simulink model "vehicle_model_cfeng"  (R2024b)
settings: Solver=FixedStepAuto  StartTime=0.0  StopTime=500.0  FixedStep=ts  RelTol=1e-3
InitFcn:
  | vehicle_parameter_Mercedes_A180
values from neighbouring files (symbols this model uses):
  acc_motor = [0, 0.13, 6.25, 12.5, 18.75, 25, 31.25, 37.5, 43.75, 50, 56.25, 62.5, 68.75, 75, 81.25, 90.63, 100]    [vehicle_parameter_Mercedes_A180.m]
  c_whl = 2 * pi * r_whl    (= 2.0106192983)    [vehicle_parameter_Mercedes_A180.m]
  eng_trq = [0, 25, 50, 75, 100, 125, 150, 175, 200, 225, 250, 275, 300]    [vehicle_parameter_Mercedes_A180.m]
  g = 9.81    [vehicle_parameter_Mercedes_A180.m]
  gear_ratios_to_neutral = [1, 1.0526, 1.1368, 1.2421, 1.3263, 1.4737, 1.6421, 1.1895]    [vehicle_parameter_Mercedes_A180.m]
  i_brems = 12    [vehicle_parameter_Mercedes_A180.m]
  m_tot = m_veh + m_pay    (= 1445)    [vehicle_parameter_Mercedes_A180.m]
  mu_brems = 0.8    [vehicle_parameter_Mercedes_A180.m]
  n_brems = 2    [vehicle_parameter_Mercedes_A180.m]
  r_air = cw_drag * A_face    (= 0.594)    [vehicle_parameter_Mercedes_A180.m]
  r_axle = 3.35    [vehicle_parameter_Mercedes_A180.m]
  r_brems = 0.1    [vehicle_parameter_Mercedes_A180.m]
  r_gear = [0.00, 4.31, 2.44, 1.35, 0.94, 0.82, 0.70, 3.38]    [vehicle_parameter_Mercedes_A180.m]
  r_roll = 0.0125    [vehicle_parameter_Mercedes_A180.m]
  r_whl = 0.32    [vehicle_parameter_Mercedes_A180.m]
  roh_air = 1.204    [vehicle_parameter_Mercedes_A180.m]
  rpm_drag = [0, 1, 500, 1000, 1500, 2000, 2500, 3000, 3500, 4000, 4500, 5000, 5500]    [vehicle_parameter_Mercedes_A180.m]
  rpm_loss = [0, 500, 1000, 1500, 2000, 2500, 3000, 3500, 4000, 4500, 5000, 5500]    [vehicle_parameter_Mercedes_A180.m]
  rpm_motor = [0, 608, 640, 736, 800, 992, 1248, 1504, 1760, 2016, 2240, 2496, 2752, 3008, 3264, 3488, 3744, 4000, 4512, 4992, 5248, 5500]    [vehicle_parameter_Mercedes_A180.m]
  torque_drag = [0, 10.27, 10.53, 10.93, 11.46, 12.12, 12.91, 13.84, 14.90, 16.09, 17.41, 18.86, 20.45]    [vehicle_parameter_Mercedes_A180.m]
  torque_loss = [ ... (first row only)    [vehicle_parameter_Mercedes_A180.m]
  torque_motor = [ ... (first row only)    [vehicle_parameter_Mercedes_A180.m]
undefined symbols (not defined in the file or in its folder): magnitude
libraries: simulink x4, slpidlib x1
settings Model: Creator=ASUS  LastModifiedBy=ASUS
settings RTWCC: GPUComputeCapability=3.5

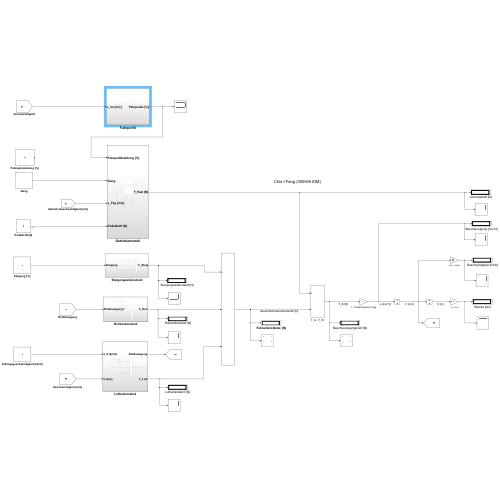
[thumbnail: Simulink's stored preview of the top-level diagram]
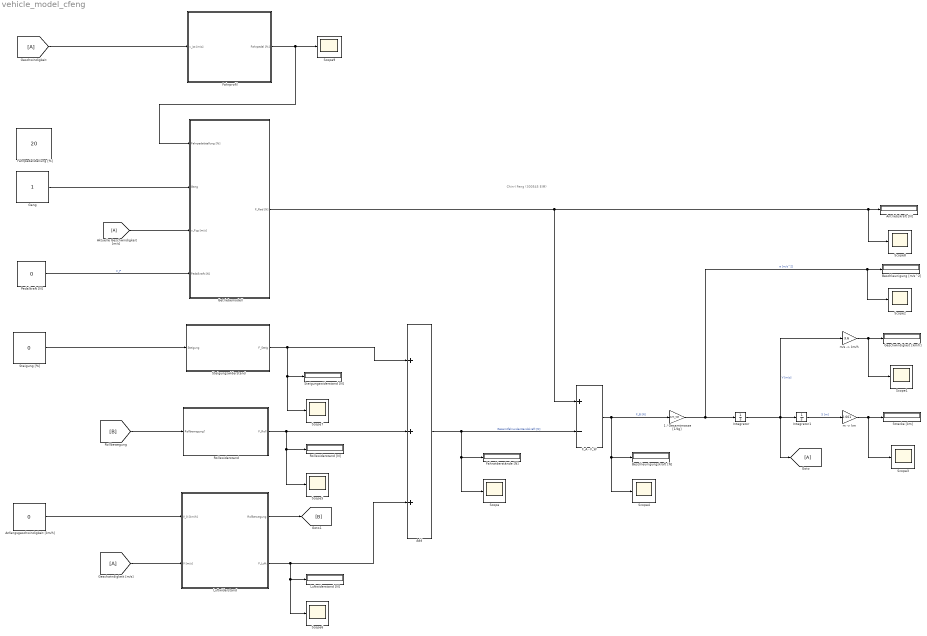
== system vehicle_model_cfeng ==
  note: Chin-I Feng (300545 EIM)
  1 / Gesamtmasse [1/kg] : Gain  Gain=1/m_tot
  Add : Sum  Inputs=+++
  Aktuelle Geschwindigkeit [m/s] : From
  Anfangsgeschwindigkeit [km/h] : Constant  Value=0  SampleTime=1
  Antriebskraft [N] : Display
  Beschleunigung [m/s^2] : Display
  Beschleunigungskraft [N] : Display
  F_A - F_W : Sum  Inputs=+-
  Fahrpedalstellung [%] : Constant  Value=20  SampleTime=1
  Fahrprofil : Subsystem
  Fahrwiderstände [N] : Display
  Gang : Constant  SampleTime=1
  Geschwindigkeit : From
  Geschwindigkeit [km/h] : Display
  Geschwindigkeit [m/s] : From
  Getriebemodell : Subsystem
  Goto : Goto
  Integrator : Integrator
  Integrator1 : Integrator
  Luftwiderstand : Subsystem
  "Luftwiderstand [N] " : Display
  Pedalkraft [N] : Constant  Value=0  SampleTime=1
  Rollswiderstand : Subsystem
  Rollswiderstand [N] : Display
  Scope{,1..9} (10 alike) : Scope
  Steigung [%] : Constant  Value=0  SampleTime=1
  Steigungswiderstand : Subsystem
  Steigungswiderstand [N] : Display
  Strecke [km] : Display
  "m -> km" : Gain  Gain=0.001
  "m/s -> km/h" : Gain  Gain=3.6
  wires:
  Add/1 -> Scope/1, Fahrwiderstände [N]/1, F_A - F_W/2  "Gesamtfahrwiderstandskraft [N]"
  F_A - F_W/1 -> Scope4/1, Beschleunigungskraft [N]/1, 1 / Gesamtmasse [1/kg]/1  "F_B [N]"
  1 / Gesamtmasse [1/kg]/1 -> Integrator/1, Scope2/1, Beschleunigung [m/s^2]/1  "a [m/s^2]"
  Integrator/1 -> "m/s -> km/h"/1, Goto/1, Integrator1/1  "V [m/s]"
  "m/s -> km/h"/1 -> Scope1/1, Geschwindigkeit [km/h]/1
  Integrator1/1 -> "m -> km"/1  "S [m]"
  "m -> km"/1 -> Scope3/1, Strecke [km]/1
  Luftwiderstand/2(F_Luft) -> "Luftwiderstand [N] "/1, Scope6/1, Add/3
  Anfangsgeschwindigkeit [km/h]/1 -> Luftwiderstand/1(V_0 [km/h])
  Steigungswiderstand/1(F_Steig) -> Add/1, Scope7/1, Steigungswiderstand [N]/1
  Rollswiderstand/1(F_Roll) -> Add/2, Scope5/1, Rollswiderstand [N]/1
  Steigung [%]/1 -> Steigungswiderstand/1(Steigung)
  Geschwindigkeit [m/s]/1 -> Luftwiderstand/2(V [m/s])
  Luftwiderstand/1(Rollbewegung) -> [B]
  [B] -> Rollswiderstand/1(Rollbewegung?)
  Getriebemodell/1(F_Rad [N]) -> F_A - F_W/1, Scope8/1, Antriebskraft [N]/1
  Gang/1 -> Getriebemodell/2(Gang)
  Aktuelle Geschwindigkeit [m/s]/1 -> Getriebemodell/3(v_Fzg [m/s])
  Geschwindigkeit/1 -> Fahrprofil/1(v_ist [m/s])
  Fahrprofil/1(Fahrpedal [%]) -> Getriebemodell/1(Fahrpedalstellung [%]), Scope9/1
  Pedalkraft [N]/1 -> Getriebemodell/4(Pedalkraft [N])  "F_P"

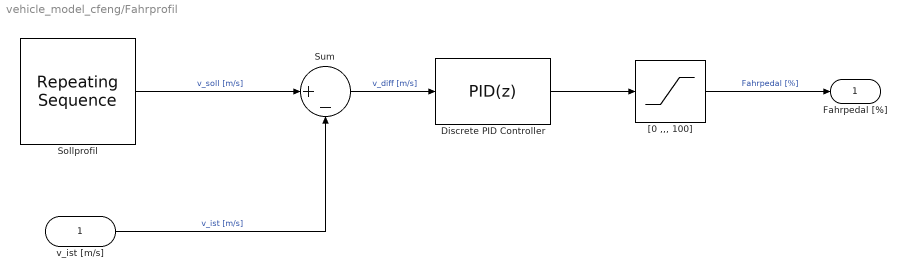
== system vehicle_model_cfeng/Fahrprofil ==
  v_ist [m/s] : Inport
  Discrete PID Controller : slpidlib/PID Controller  Controller=PID  Form=Parallel  TimeDomain=Discrete-time  UseExternalTs=off  SampleTime=-1  IntegratorMethod=Forward Euler  FilterMethod=Forward Euler  ControllerParametersSource=internal  P=1  I=1  UseKiTs=off  D=0  UseExternalDerivativeSource=off  N=100  UseFilter=on  TunerSelectOption=Transfer Function Based (PID Tuner App)  InitialConditionSource=internal  InitialConditionForIntegrator=0  InitialConditionForFilter=0  DifferentiatorICPrevScaledInput=0  ExternalReset=none  TrackingMode=off  Kt=1  LimitOutput=off  SatLimitsSource=internal  UpperSaturationLimit=inf  LowerSaturationLimit=-inf  LinearizeAsGain=off  AntiWindupMode=none  Kb=1  LimitIntegrator=off  UpperIntegratorSaturationLimit=inf  LowerIntegratorSaturationLimit=-inf  POutMin=[]  POutMax=[]  IOutMin=[]  IOutMax=[]  DOutMin=[]  DOutMax=[]  NOutMin=[]  NOutMax=[]  SumOutMin=[]  SumOutMax=[]  SaturationOutMin=[]  SaturationOutMax=[]  PParamMin=[]  PParamMax=[]  IParamMin=[]  IParamMax=[]  DParamMin=[]  DParamMax=[]  NParamMin=[]  NParamMax=[]  KbParamMin=[]  KbParamMax=[]  KtParamMin=[]  KtParamMax=[]  KbOutMin=[]  KbOutMax=[]  KtOutMin=[]  KtOutMax=[]  IntegratorOutMin=[]  IntegratorOutMax=[]  FilterOutMin=[]  FilterOutMax=[]  SumI1OutMin=[]  SumI1OutMax=[]  SumI2OutMin=[]  SumI2OutMax=[]  SumI3OutMin=[]  SumI3OutMax=[]  SumI4OutMin=[]  SumI4OutMax=[]  SumDOutMin=[]  SumDOutMax=[]  DifferentiatorOutMin=[]  DifferentiatorOutMax=[]  FilterDiffOutCoefMin=[]  FilterDiffOutCoefMax=[]  ReciprocalOutMin=[]  ReciprocalOutMax=[]  SumDenOutMin=[]  SumDenOutMax=[]  SumNumOutMin=[]  SumNumOutMax=[]  DivideOutMin=[]  DivideOutMax=[]  UdiffTsProdOutMin=[]  UdiffTsProdOutMax=[]  NTsProdOutMin=[]  NTsProdOutMax=[]  UintegralTsProdOutMin=[]  UintegralTsProdOutMax=[]  UngainTsProdOutMin=[]  UngainTsProdOutMax=[]  ClampingZeroOutDataTypeStr=Inherit: Inherit via back propagation  ClampingZeroOutMin=[]  ClampingZeroOutMax=[]  FilterDenConstantOutDataTypeStr=Inherit: Inherit via back propagation  FilterDenConstantOutMin=[]  FilterDenConstantOutMax=[]  PCopyOutDataTypeStr=Inherit: Inherit via back propagation  PCopyOutMin=[]  PCopyOutMax=[]  NCopyOutDataTypeStr=Inherit: Inherit via back propagation  NCopyOutMin=[]  NCopyOutMax=[]  IntegratorContinuousStateAttributes=''  IntegratorStateMustResolveToSignalObject=off  IntegratorRTWStateStorageClass=Auto  FilterContinuousStateAttributes=''  FilterStateMustResolveToSignalObject=off  FilterRTWStateStorageClass=Auto  ParallelPVariant=InternalParameters  IdealPVariant=Disabled  IVariant=InternalParameters  DVariant=InternalParameters  IntegratorVariant=Discrete  SatVariant=Disabled  AWVariant=Passthrough  PCopyVariant=Disabled  TRVariant=Disabled  FdbkBlocksVariant=Forward  IdealPFdbkVariant=Disabled  SatFdbkVariant=Disabled  DerivativeFilterVariant=ForwardEulerFilter  NVariant=InternalParameters  NCopyVariant=Disabled  FilterICVariant=InternalICsFilter  IntegratorICVariant=InternalICs  ExternalResetVariant=Disabled  TRSumVariant=Passthrough  SumFdbkVariant=Disabled  SumVariant=Sum_PID  TsampFilterVariant=InternalTs  TsampNgainVariant=Passthrough  TsampIntegralVariant=Disabled_SignalSpec  ExternalSaturationOutDataTypeStr=Inherit: Same as second input  DerivativeSourceVariant=ErrorSignal  PreIntVariant=InternalPreInt
      settings: LibrarySourceBlock=simulink/Discrete/Discrete PID Controller
  Sollprofil : simulink/Sources/Repeating Sequence  rep_seq_t=[0 50 100 1100 1150 1200]  rep_seq_y=[0 0 27 44 0 0]
  Sum : Sum  Inputs=|+-
  "[0 ,,, 100]" : Saturate  UpperLimit=100  LowerLimit=0
  Fahrpedal [%] : Outport
  wires:
  "[0 ,,, 100]"/1 -> Fahrpedal [%]/1  "Fahrpedal [%]"
  Sum/1 -> Discrete PID Controller/1  "v_diff [m/s]"
  Sollprofil/1 -> Sum/1  "v_soll [m/s]"
  Discrete PID Controller/1 -> "[0 ,,, 100]"/1
  v_ist [m/s]/1 -> Sum/2  "v_ist [m/s]"

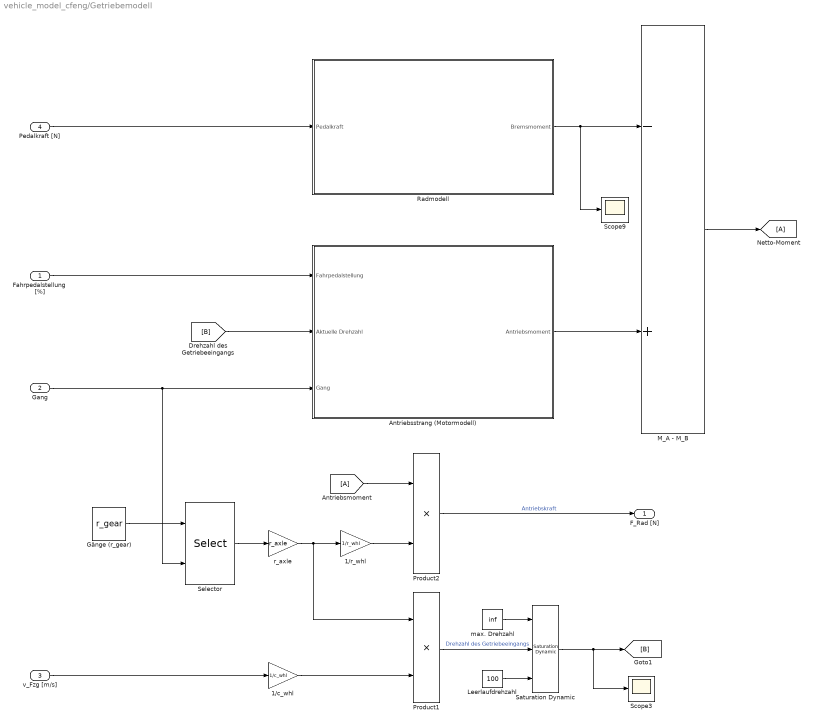
== system vehicle_model_cfeng/Getriebemodell ==
  Fahrpedalstellung [%] : Inport
  Gang : Inport  Port=2
  v_Fzg [m/s] : Inport  Port=3
  Pedalkraft [N] : Inport  Port=4
  1/c_whl : Gain  Gain=1/c_whl
  1/r_whl : Gain  Gain=1/r_whl
  Antriebsmoment : From
  Antriebsstrang (Motormodell) : Subsystem
  Gänge (r_gear) : Constant  Value=r_gear  SampleTime=1
  Leerlaufdrehzahl : Constant  Value=100  SampleTime=1
  M_A - M_B : Sum  Inputs=-+
  Netto-Moment : Goto
  Product1 : Product
  Product2 : Product
  Radmodell : Subsystem
  Saturation Dynamic : simulink/Discontinuities/Saturation Dynamic  OutMin=[]  OutMax=[]  OutDataTypeStr=Inherit: Same as second input  OutDataType=fixdt(1, 16)  OutScaling=2^-10  DoSatur=off
  Scope3 : Scope
  Scope9 : Scope
  Selector : Selector  IndexMode=Zero-based  InputPortWidth=8  IndexOptions=Index vector (port)  Indices=1  OutputSizes=1
  max. Drehzahl : Constant  Value=inf  SampleTime=1
  r_axle : Gain  Gain=r_axle
  F_Rad [N] : Outport
  wires:
  Product2/1 -> F_Rad [N]/1  "Antriebskraft"
  r_axle/1 -> Product1/1, 1/r_whl/1
  Selector/1 -> r_axle/1
  Gang/1 -> Selector/2, Antriebsstrang (Motormodell)/3(Gang)
  Gänge (r_gear)/1 -> Selector/1
  1/r_whl/1 -> Product2/2
  Product1/1 -> Saturation Dynamic/2  "Drehzahl des Getriebeeingangs"
  v_Fzg [m/s]/1 -> 1/c_whl/1
  1/c_whl/1 -> Product1/2
  max. Drehzahl/1 -> Saturation Dynamic/1
  Leerlaufdrehzahl/1 -> Saturation Dynamic/3
  Saturation Dynamic/1 -> [B], Scope3/1
  Fahrpedalstellung [%]/1 -> Antriebsstrang (Motormodell)/1(Fahrpedalstellung)
  Antriebsmoment/1 -> Product2/1
  [B] -> Antriebsstrang (Motormodell)/2(Aktuelle Drehzahl)
  Antriebsstrang (Motormodell)/1("Antriebsmoment ") -> M_A - M_B/2
  M_A - M_B/1 -> Netto-Moment/1
  Radmodell/1(Bremsmoment) -> Scope9/1, M_A - M_B/1
  Pedalkraft [N]/1 -> Radmodell/1(Pedalkraft)

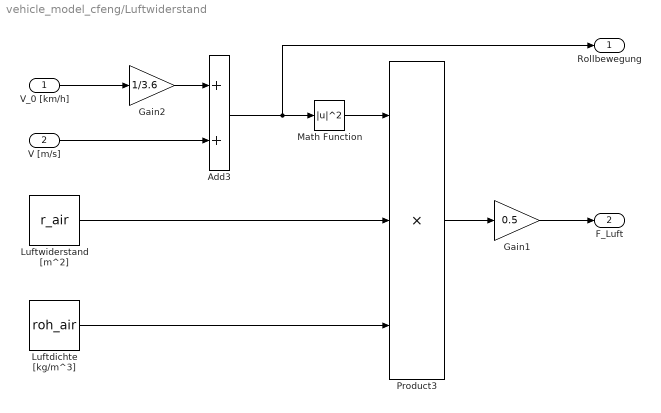
== system vehicle_model_cfeng/Luftwiderstand ==
  V_0 [km/h] : Inport
  V [m/s] : Inport  Port=2
  Add3 : Sum
  Gain1 : Gain  Gain=0.5
  Gain2 : Gain  Gain=1/3.6
  Luftdichte [kg/m^3] : Constant  Value=roh_air  SampleTime=1
  Luftwiderstand [m^2] : Constant  Value=r_air  SampleTime=1
  Math Function : Math  Operator=magnitude^2
  Product3 : Product  Inputs=3
  Rollbewegung : Outport
  F_Luft : Outport  Port=2
  wires:
  Gain2/1 -> Add3/1
  V [m/s]/1 -> Add3/2
  Luftwiderstand [m^2]/1 -> Product3/2
  Luftdichte [kg/m^3]/1 -> Product3/3
  Add3/1 -> Rollbewegung/1, Math Function/1
  Product3/1 -> Gain1/1
  Math Function/1 -> Product3/1
  Gain1/1 -> F_Luft/1
  V_0 [km/h]/1 -> Gain2/1

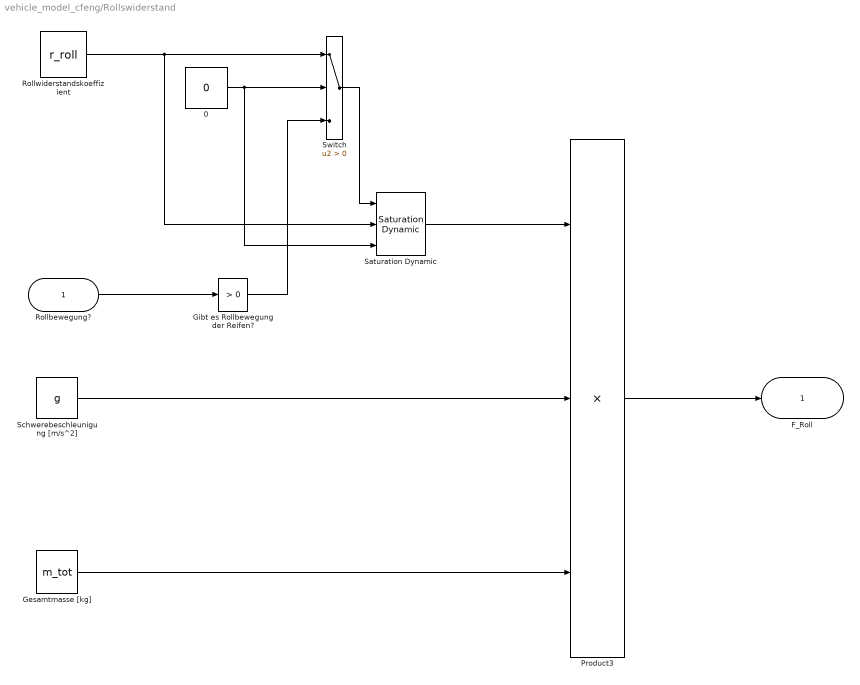
== system vehicle_model_cfeng/Rollswiderstand ==
  Rollbewegung? : Inport
  0 : Constant  Value=0  SampleTime=1
  Gesamtmasse [kg] : Constant  Value=m_tot  SampleTime=1
  Gibt es Rollbewegung der Reifen? : simulink/Logic and Bit Operations/Compare To Constant  relop=>  const=0  OutDataTypeStr=uint8
  Product3 : Product  Inputs=3
  Rollwiderstandskoeffizient : Constant  Value=r_roll  SampleTime=1
  Saturation Dynamic : simulink/Discontinuities/Saturation Dynamic  OutMin=[]  OutMax=[]  OutDataTypeStr=Inherit: Same as second input  OutDataType=fixdt(1, 16)  OutScaling=2^-10  DoSatur=off
  Schwerebeschleunigung [m/s^2] : Constant  Value=g  SampleTime=1
  Switch : Switch  Criteria=u2 > Threshold  SaturateOnIntegerOverflow=off  InputSameDT=off
  F_Roll : Outport
  wires:
  Saturation Dynamic/1 -> Product3/1
  Gesamtmasse [kg]/1 -> Product3/3
  Schwerebeschleunigung [m/s^2]/1 -> Product3/2
  0/1 -> Saturation Dynamic/3, Switch/2
  Switch/1 -> Saturation Dynamic/1
  Rollwiderstandskoeffizient/1 -> Saturation Dynamic/2, Switch/1
  Product3/1 -> F_Roll/1
  Gibt es Rollbewegung der Reifen?/1 -> Switch/3
  Rollbewegung?/1 -> Gibt es Rollbewegung der Reifen?/1

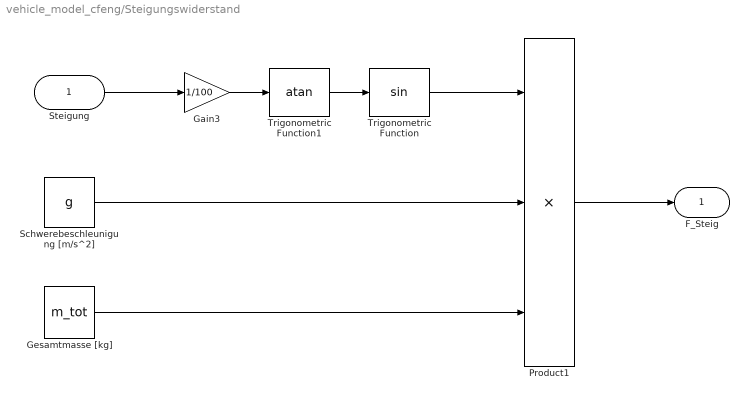
== system vehicle_model_cfeng/Steigungswiderstand ==
  Steigung : Inport
  Gain3 : Gain  Gain=1/100
  Gesamtmasse [kg] : Constant  Value=m_tot  SampleTime=1
  Product1 : Product  Inputs=3
  Schwerebeschleunigung [m/s^2] : Constant  Value=g  SampleTime=1
  Trigonometric Function : Trigonometry
  Trigonometric Function1 : Trigonometry  Operator=atan
  F_Steig : Outport
  wires:
  Gesamtmasse [kg]/1 -> Product1/3
  Gain3/1 -> Trigonometric Function1/1
  Trigonometric Function1/1 -> Trigonometric Function/1
  Trigonometric Function/1 -> Product1/1
  Schwerebeschleunigung [m/s^2]/1 -> Product1/2
  Product1/1 -> F_Steig/1
  Steigung/1 -> Gain3/1

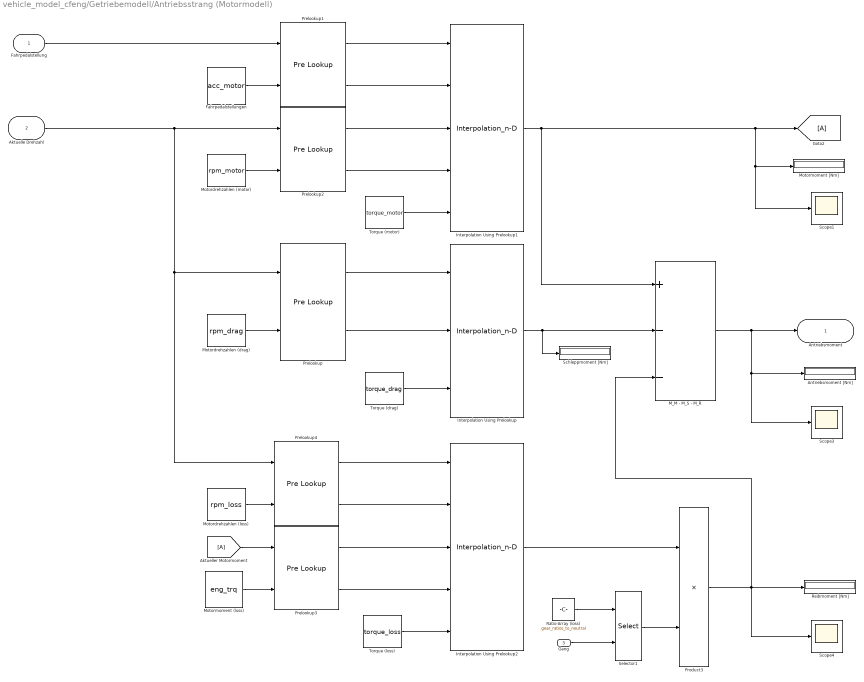
== system vehicle_model_cfeng/Getriebemodell/Antriebsstrang (Motormodell) ==
  Fahrpedalstellung : Inport
  Aktuelle Drehzahl : Inport  Port=2
  Gang : Inport  Port=3
  Aktueller Motormoment : From
  Antriebsmoment [Nm] : Display
  Fahrpedalstellungen : Constant  Value=acc_motor  SampleTime=1
  Goto2 : Goto
  Interpolation Using Prelookup : Interpolation_n-D  NumberOfTableDimensions=1  TableSource=Input port  ValidIndexMayReachLast=on  InternalRulePriority=Speed
      settings: InputPortMap=u0,u1,p2
  Interpolation Using Prelookup1 : Interpolation_n-D  TableSource=Input port  InternalRulePriority=Speed
      settings: InputPortMap=u0,u1,u2,u3,p2
  Interpolation Using Prelookup2 : Interpolation_n-D  TableSource=Input port  InternalRulePriority=Speed
      settings: InputPortMap=u0,u1,u2,u3,p2
  M_M - M_S - M_R : Sum  Inputs=+--
  Motordrehzahlen (drag) : Constant  Value=rpm_drag  SampleTime=1
  Motordrehzahlen (loss) : Constant  Value=rpm_loss  SampleTime=1
  Motordrehzahlen (motor) : Constant  Value=rpm_motor  SampleTime=1
  Motormoment (loss) : Constant  Value=eng_trq  SampleTime=1
  Motormoment [Nm] : Display
  Prelookup : PreLookup  BreakpointsDataSource=Input port  BreakpointsData=[10:10:110]  BeginIndexSearchUsingPreviousIndexResult=on  ExtrapMethod=Linear
      settings: InputPortMap=u0,p1
  Prelookup1 : PreLookup  BreakpointsDataSource=Input port  BreakpointsData=[10:10:110]  BeginIndexSearchUsingPreviousIndexResult=on  UseLastBreakpoint=on
      settings: InputPortMap=u0,p1
  Prelookup2 : PreLookup  BreakpointsDataSource=Input port  BreakpointsData=[10:10:110]  BeginIndexSearchUsingPreviousIndexResult=on
      settings: InputPortMap=u0,p1
  Prelookup3 : PreLookup  BreakpointsDataSource=Input port  BreakpointsData=[10:10:110]  BeginIndexSearchUsingPreviousIndexResult=on  UseLastBreakpoint=on
      settings: InputPortMap=u0,p1
  Prelookup4 : PreLookup  BreakpointsDataSource=Input port  BreakpointsData=[10:10:110]  BeginIndexSearchUsingPreviousIndexResult=on  UseLastBreakpoint=on
      settings: InputPortMap=u0,p1
  Product3 : Product
  Ratio-Array (loss) : Constant  Value=gear_ratios_to_neutral  SampleTime=1
  Reibmoment [Nm] : Display
  Schleppmoment [Nm] : Display
  Scope1 : Scope
  Scope3 : Scope
  Scope4 : Scope
  Selector1 : Selector  IndexMode=Zero-based  InputPortWidth=8  IndexOptions=Index vector (port)  Indices=1  OutputSizes=1
  Torque (drag) : Constant  Value=torque_drag  SampleTime=1
  Torque (loss) : Constant  Value=torque_loss  SampleTime=1
  Torque (motor) : Constant  Value=torque_motor  SampleTime=1
  "Antriebsmoment " : Outport
  wires:
  Prelookup2/1 -> Interpolation Using Prelookup1/3
  Torque (motor)/1 -> Interpolation Using Prelookup1/5
  Prelookup/2 -> Interpolation Using Prelookup/2
  Motordrehzahlen (drag)/1 -> Prelookup/2
  Prelookup/1 -> Interpolation Using Prelookup/1
  Prelookup1/1 -> Interpolation Using Prelookup1/1
  Prelookup1/2 -> Interpolation Using Prelookup1/2
  Fahrpedalstellungen/1 -> Prelookup1/2
  Prelookup2/2 -> Interpolation Using Prelookup1/4
  Torque (drag)/1 -> Interpolation Using Prelookup/3
  Motordrehzahlen (motor)/1 -> Prelookup2/2
  Interpolation Using Prelookup1/1 -> M_M - M_S - M_R/1, Scope1/1, Motormoment [Nm]/1, Goto2/1
  M_M - M_S - M_R/1 -> "Antriebsmoment "/1, Antriebsmoment [Nm]/1, Scope3/1
  Fahrpedalstellung/1 -> Prelookup1/1
  Interpolation Using Prelookup/1 -> M_M - M_S - M_R/2, Schleppmoment [Nm]/1
  Aktuelle Drehzahl/1 -> Prelookup4/1, Prelookup/1, Prelookup2/1
  Aktueller Motormoment/1 -> Prelookup3/1
  Motormoment (loss)/1 -> Prelookup3/2
  Prelookup4/1 -> Interpolation Using Prelookup2/1
  Prelookup4/2 -> Interpolation Using Prelookup2/2
  Prelookup3/1 -> Interpolation Using Prelookup2/3
  Prelookup3/2 -> Interpolation Using Prelookup2/4
  Torque (loss)/1 -> Interpolation Using Prelookup2/5
  Motordrehzahlen (loss)/1 -> Prelookup4/2
  Interpolation Using Prelookup2/1 -> Product3/1
  Ratio-Array (loss)/1 -> Selector1/1
  Gang/1 -> Selector1/2
  Selector1/1 -> Product3/2
  Product3/1 -> Scope4/1, M_M - M_S - M_R/3, Reibmoment [Nm]/1

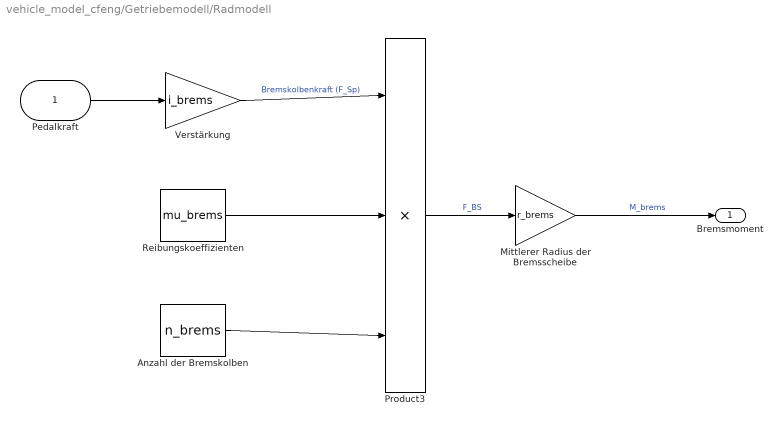
== system vehicle_model_cfeng/Getriebemodell/Radmodell ==
  Pedalkraft : Inport
  Anzahl der Bremskolben : Constant  Value=n_brems  SampleTime=1
  Mittlerer Radius der Bremsscheibe : Gain  Gain=r_brems
  Product3 : Product  Inputs=3
  Reibungskoeffizienten : Constant  Value=mu_brems  SampleTime=1
  Verstärkung : Gain  Gain=i_brems
  Bremsmoment : Outport
  wires:
  Anzahl der Bremskolben/1 -> Product3/3
  Product3/1 -> Mittlerer Radius der Bremsscheibe/1  "F_BS"
  Reibungskoeffizienten/1 -> Product3/2
  Verstärkung/1 -> Product3/1  "Bremskolbenkraft (F_Sp)"
  Mittlerer Radius der Bremsscheibe/1 -> Bremsmoment/1  "M_brems"
  Pedalkraft/1 -> Verstärkung/1
